simulink model "V2V_Simulation"  (R2025b)
settings: Solver=ode45  StartTime=0.0  StopTime=10  MaxStep=0.01  RelTol=1e-3
settings Model: Creator=suraj  LastModifiedBy=suraj

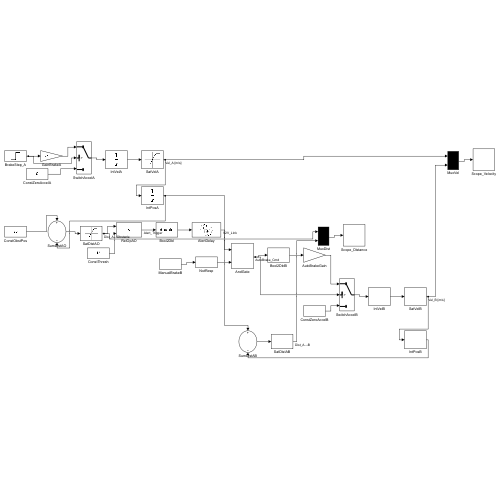
[thumbnail: Simulink's stored preview of the top-level diagram]
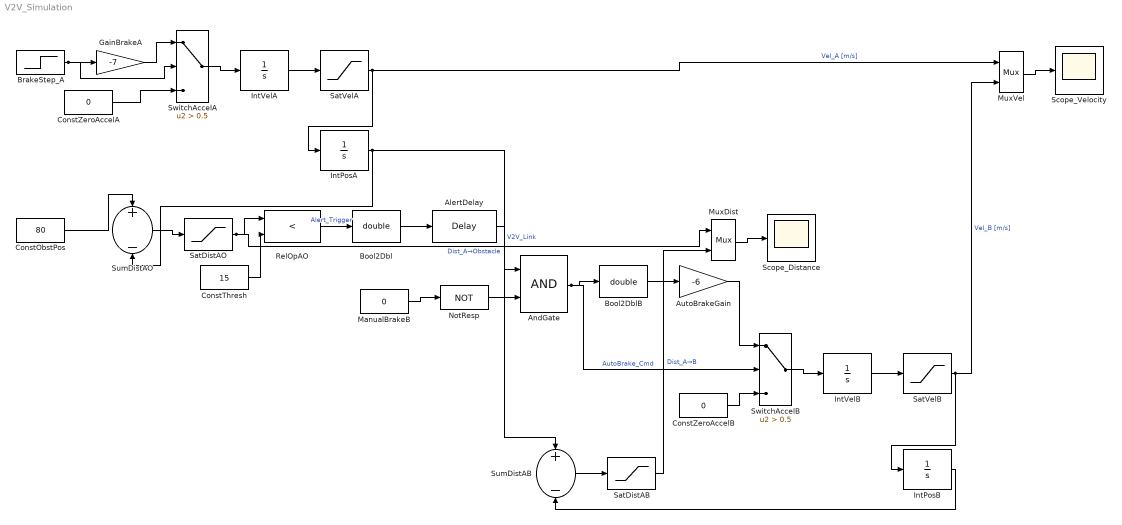
== system V2V_Simulation ==
  AlertDelay : TransportDelay  DelayTime=0.2
  AndGate : Logic  AllPortsSameDT=off  OutDataTypeStr=boolean
  AutoBrakeGain : Gain  Gain=-6
  Bool2Dbl : DataTypeConversion  OutDataTypeStr=double  SaturateOnIntegerOverflow=off  RndMeth=Floor
  Bool2DblB : DataTypeConversion  OutDataTypeStr=double  SaturateOnIntegerOverflow=off  RndMeth=Floor
  BrakeStep_A : Step  Time=2.5  SampleTime=0
  ConstObstPos : Constant  Value=80
  ConstThresh : Constant  Value=15
  ConstZeroAccelA : Constant  Value=0
  ConstZeroAccelB : Constant  Value=0
  GainBrakeA : Gain  Gain=-7
  IntPosA : Integrator
  IntPosB : Integrator  InitialCondition=-15
  IntVelA : Integrator  InitialCondition=20
  IntVelB : Integrator  InitialCondition=20
  ManualBrakeB : Constant  Value=0
  MuxDist : Mux  Inputs=2
  MuxVel : Mux  Inputs=2
  NotResp : Logic  Operator=NOT  AllPortsSameDT=off  OutDataTypeStr=boolean
  RelOpAO : RelationalOperator  Operator=<  OutDataTypeStr=boolean  RndMeth=Simplest  InputSameDT=off
  SatDistAB : Saturate  UpperLimit=200  LowerLimit=0
  SatDistAO : Saturate  UpperLimit=200  LowerLimit=0
  SatVelA : Saturate  UpperLimit=100  LowerLimit=0
  SatVelB : Saturate  UpperLimit=100  LowerLimit=0
  Scope_Distance : Scope
      settings: TimeSpan=10  Title=Distances — A→Obstacle (ch1), A→B (ch2)  YLabel=Distance (m)
  Scope_Velocity : Scope
      settings: TimeSpan=10  Title=Vehicle Velocities — A (ch1) vs B (ch2)  YLabel=Velocity (m/s)
  SumDistAB : Sum  Inputs=+-
  SumDistAO : Sum  Inputs=+-
  SwitchAccelA : Switch  Criteria=u2 > Threshold  Threshold=0.5  SaturateOnIntegerOverflow=off  InputSameDT=off
  SwitchAccelB : Switch  Criteria=u2 > Threshold  Threshold=0.5  SaturateOnIntegerOverflow=off  InputSameDT=off
  wires:
  BrakeStep_A/1 -> GainBrakeA/1, SwitchAccelA/2
  GainBrakeA/1 -> SwitchAccelA/1
  ConstZeroAccelA/1 -> SwitchAccelA/3
  SwitchAccelA/1 -> IntVelA/1
  IntVelA/1 -> SatVelA/1
  SatVelA/1 -> IntPosA/1, MuxVel/1  "Vel_A [m/s]"
  ConstObstPos/1 -> SumDistAO/1
  IntPosA/1 -> SumDistAO/2, SumDistAB/1
  SumDistAO/1 -> SatDistAO/1
  SatDistAO/1 -> RelOpAO/1, MuxDist/1  "Dist_A→Obstacle"
  ConstThresh/1 -> RelOpAO/2
  RelOpAO/1 -> Bool2Dbl/1  "Alert_Trigger"
  Bool2Dbl/1 -> AlertDelay/1
  AlertDelay/1 -> AndGate/1  "V2V_Link"
  ManualBrakeB/1 -> NotResp/1
  NotResp/1 -> AndGate/2
  AndGate/1 -> Bool2DblB/1, SwitchAccelB/2  "AutoBrake_Cmd"
  Bool2DblB/1 -> AutoBrakeGain/1
  AutoBrakeGain/1 -> SwitchAccelB/1
  ConstZeroAccelB/1 -> SwitchAccelB/3
  SwitchAccelB/1 -> IntVelB/1
  IntVelB/1 -> SatVelB/1
  SatVelB/1 -> IntPosB/1, MuxVel/2  "Vel_B [m/s]"
  IntPosB/1 -> SumDistAB/2
  SumDistAB/1 -> SatDistAB/1
  MuxVel/1 -> Scope_Velocity/1
  SatDistAB/1 -> MuxDist/2  "Dist_A→B"
  MuxDist/1 -> Scope_Distance/1
